simulink model "BlockedRotorTest"  (R2019b)
settings: Solver=ode23tb  StartTime=0.0  StopTime=15  RelTol=1e-3
undefined symbols (not defined in the file): f, ftest, LrDash, Ls, P, RrDash, Rs, VLL, Vpeak
libraries: powerlib x11, powerlib_meascontrol x5
settings Model: Creator=FAST  LastModifiedBy=FAST

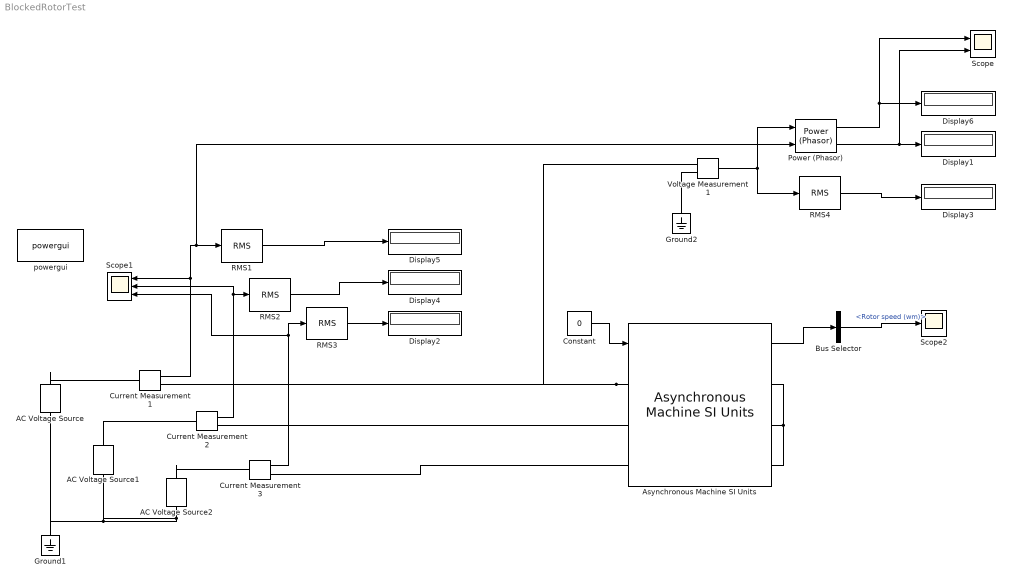
== system BlockedRotorTest ==
  AC Voltage Source : powerlib/Electrical Sources/AC Voltage Source  Amplitude=Vpeak  Phase=0  Frequency=ftest  SampleTime=0  Measurements=None  BusType=swing  Pref=10e3  Qref=0  Qmin=-inf  Qmax=+inf
      settings: SourceProductName=Simscape Electrical
  AC Voltage Source1 : powerlib/Electrical Sources/AC Voltage Source  Amplitude=Vpeak  Phase=120  Frequency=ftest  SampleTime=0  Measurements=None  BusType=swing  Pref=10e3  Qref=0  Qmin=-inf  Qmax=+inf
      settings: SourceProductName=Simscape Electrical
  AC Voltage Source2 : powerlib/Electrical Sources/AC Voltage Source  Amplitude=Vpeak  Phase=240  Frequency=ftest  SampleTime=0  Measurements=None  BusType=swing  Pref=10e3  Qref=0  Qmin=-inf  Qmax=+inf
      settings: SourceProductName=Simscape Electrical
  Asynchronous Machine SI Units : powerlib/Machines/Asynchronous Machine SI Units  RotorType=Wound  PresetModel=No  MechanicalLoad=Torque Tm  ShowDetailedParameters=on  ReferenceFrame=Rotor  Units=SI  MeasurementBus=off  NominalParameters=[P VLL f]  Stator=[Rs Ls]  Rotor=[RrDash LrDash]  Cage1=[0.4155 0.002066]  Cage2=[0.4168 0.0003495]  Lm=Lm  Mechanical=[0.05 0.005879 2]  PolePairs=2  InitialConditions=[0 0 0 0 0 0 0 0]  SimulateSaturation=off  Saturation=[14.03593122, 27.81365428, 53.79336849, 72.68890987, 97.98006896, 148.6815601, 215.7428561, 302.9841135, 428.7778367 ; 230, 322, 414, 460, 506, 552, 598, 644, 690]  LoadFlowParameters=1492000  TsPowergui=0  TsBlock=-1  IterativeModel=Trapezoidal non iterative  IterativeDiscreteModel=Trapezoidal non iterative  Pmec=1.492e+006
      settings: SourceProductName=Simscape Electrical
  Bus Selector : BusSelector  OutputSignals=Mechanical.Rotor speed (wm)
  Constant : Constant  Value=0
  Current Measurement1 : powerlib/Measurements/Current Measurement  PhasorSimulation=off  OutputType=Complex  PSBequivalent=0
      settings: SourceProductName=Simscape Electrical
  Current Measurement2 : powerlib/Measurements/Current Measurement  PhasorSimulation=off  OutputType=Complex  PSBequivalent=0
      settings: SourceProductName=Simscape Electrical
  Current Measurement3 : powerlib/Measurements/Current Measurement  PhasorSimulation=off  OutputType=Complex  PSBequivalent=0
      settings: SourceProductName=Simscape Electrical
  Display{1..6} (6 alike) : Display
  Ground1 : powerlib/Elements/Ground  LConnTagsString=a
      settings: SourceProductName=Simscape Electrical
  Ground2 : powerlib/Elements/Ground  LConnTagsString=a
      settings: SourceProductName=Simscape Electrical
  Power (Phasor) : powerlib_meascontrol/Measurements/Power (Phasor)
      settings: SourceProductName=Simscape Electrical  SourceProductBaseCode=PS
  RMS1 : powerlib_meascontrol/Measurements/RMS  TrueRMS=on  Freq=60  RMSInit=10  Ts=0
      settings: SourceProductName=Simscape Electrical
  RMS2 : powerlib_meascontrol/Measurements/RMS  TrueRMS=on  Freq=60  RMSInit=10  Ts=0
      settings: SourceProductName=Simscape Electrical
  RMS3 : powerlib_meascontrol/Measurements/RMS  TrueRMS=on  Freq=60  RMSInit=10  Ts=0
      settings: SourceProductName=Simscape Electrical
  RMS4 : powerlib_meascontrol/Measurements/RMS  TrueRMS=on  Freq=60  RMSInit=120  Ts=0
      settings: SourceProductName=Simscape Electrical
  Scope : Scope  NumInputPorts=2
  Scope1 : Scope  NumInputPorts=3
  Scope2 : Scope
  Voltage Measurement1 : powerlib/Measurements/Voltage Measurement  PhasorSimulation=off  OutputType=Complex  PSBequivalent=0
      settings: SourceProductName=Simscape Electrical
  powergui : powerlib/powergui  Priority=1  SimulationMode=Continuous  SampleTime=50e-6  frequency=60  Iterations=50  frequencyindice=60  Pbase=100e6  ErrMax=1e-4  UnitsV=kV  UnitsW=MW  buscounter=0  FunctionMessages=off  echomessages=off  EnableUseOfTLC=off  CurrentSourceSwitches=off  DisableSnubberDevices=off  DisableRonSwitches=off  DisableVfSwitches=off  DisplayEquations=off  AutomaticDiscreteSolvers=off  SolverType=Tustin/Backward Euler (TBE)  Interpol=off  ExternalGateDelay=off  methode=off  Ts=100  x0status=blocks  SPID=on  SwTol=0  HookPort=off  NonlinearTolerance=1e-4  nMaxIteration=100  ContinueOnMaxIteration=off  RestoreLinks=warning  ResistiveCurrentMeasurement=off  Frange=[0:2:500]  Ylog=off  Xlog=on  ShowGrid=off  save=off  variable=ZData  structure=0  ZoomFFT=off  StartTime=0.0  cycles=1  DisplayStyle=1  fundamental=60  FreqAxis=off  MaxFrequency=1000  frequencyindicesteady=1  RmsSteady=1  display=off
      settings: SourceProductName=Simscape Electrical
  wires:
  Current Measurement1/1 -> Power (Phasor)/2, RMS1/1, Scope1/1
  Power (Phasor)/2 -> Scope/2, Display1/1
  Bus Selector/1 -> Scope2/1  "<Rotor speed (wm)>"
  Voltage Measurement1/1 -> RMS4/1, Power (Phasor)/1
  RMS1/1 -> Display5/1
  Power (Phasor)/1 -> Scope/1, Display6/1
  Current Measurement2/1 -> Scope1/2, RMS2/1
  Constant/1 -> Asynchronous Machine SI Units/1
  Current Measurement3/1 -> Scope1/3, RMS3/1
  RMS2/1 -> Display4/1
  RMS3/1 -> Display2/1
  RMS4/1 -> Display3/1
  Asynchronous Machine SI Units/1 -> Bus Selector/1
  connections:
  AC Voltage Source2/LConn1 -- Ground1/LConn1 -- AC Voltage Source/LConn1 -- AC Voltage Source1/LConn1
  Asynchronous Machine SI Units/LConn1 -- Current Measurement1/RConn1 -- Voltage Measurement1/LConn1
  Asynchronous Machine SI Units/RConn2 -- Asynchronous Machine SI Units/RConn1 -- Asynchronous Machine SI Units/RConn3
  Current Measurement3/RConn1 -- Asynchronous Machine SI Units/LConn3
  Current Measurement2/RConn1 -- Asynchronous Machine SI Units/LConn2
  Ground2/LConn1 -- Voltage Measurement1/LConn2
  AC Voltage Source/RConn1 -- Current Measurement1/LConn1
  AC Voltage Source2/RConn1 -- Current Measurement3/LConn1
  AC Voltage Source1/RConn1 -- Current Measurement2/LConn1
